simulink model "RIO_DKin_Simul"  (R2024b)
settings: Solver=VariableStepAuto  StartTime=0.0  StopTime=inf  RelTol=1e-3  EnableMultiTasking=on
libraries: vrlib x7, simulink x6, RIO_Lib x1
settings Model: Creator=jorgemartins  LastModifiedBy=pepev
settings SolverCC: AlgebraicLoopSolver=TrustRegion
settings DataIOCC: LimitDataPoints=on  ReturnWorkspaceOutputs=off
settings OptimizationCC: LifeSpan=inf
settings DebuggingCC: UnconnectedInputMsg=warning  UnconnectedOutputMsg=warning  UnconnectedLineMsg=warning  AllowSymbolicDim=off  SFUnexpectedBacktrackingDiag=warning  SFNoUnconditionalDefaultTransitionDiag=warning  SFExecutionAtInitializationDiag=none  ArithmeticOperatorsInVariantConditions=warning
settings ModelReferenceCC: EnableRefExpFcnMdlSchedulingChecks=on  PropagateSignalLabelsOutOfModel=off
settings SFSimCC: SimUseLocalCustomCode=off  CustomCodeUndefinedFunction=UseInterfaceOnly
settings RTWCC: RTWUseLocalCustomCode=off  GPUComputeCapability=3.5
settings CodeAppCC: StateflowObjectComments=on
settings GRTTargetCC: TargetLangStandard=C89/C90 (ANSI)
settings ConfigComp: CovMetricSettings=dw  CovSaveCumulativeToWorkspaceVar=on  CovSaveSingleToWorkspaceVar=on  CovExternalEMLEnable=off

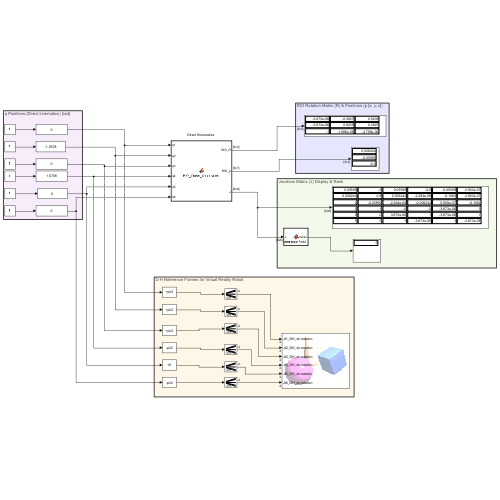
[thumbnail: Simulink's stored preview of the top-level diagram]
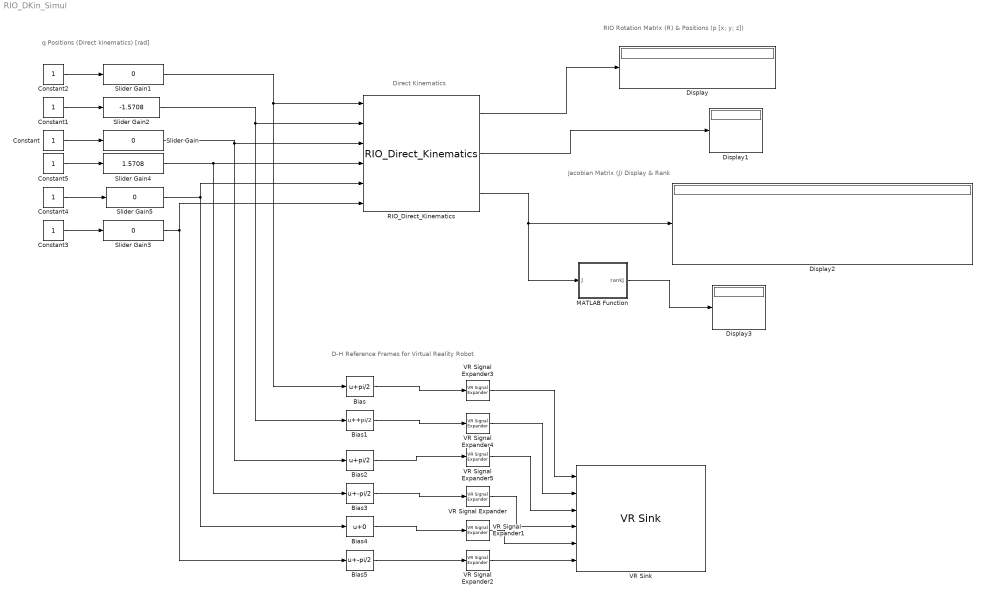
== system RIO_DKin_Simul ==
  note: Direct Kinematics
  note: D-H Reference Frames for Virtual Reality Robot
  note: Jacobian Matrix (J) Display & Rank
  note: RIO Rotation Matrix (R) & Positions (p [x; y; z])
  note: q Positions (Direct kinematics) [rad]
  Bias : Bias  Bias=pi/2  SaturateOnIntegerOverflow=off
  Bias1 : Bias  Bias=+pi/2  SaturateOnIntegerOverflow=off
  Bias2 : Bias  Bias=pi/2  SaturateOnIntegerOverflow=off
  Bias3 : Bias  Bias=-pi/2  SaturateOnIntegerOverflow=off
  Bias4 : Bias  SaturateOnIntegerOverflow=off
  Bias5 : Bias  Bias=-pi/2  SaturateOnIntegerOverflow=off
  Constant{,1..5} (6 alike) : Constant
  Display{,1..3} (4 alike) : Display
  MATLAB Function : MATLAB Function  TreatAsAtomicUnit=on
  RIO_Direct_Kinematics : RIO_Lib/RIO_Direct_Kinematics  SystemSampleTime=-1  VariantActivationTime=update diagram  AllowFlexibleInterface=on  Latency=0  AutoFrameSizeCalculation=off
  Slider Gain{,1,3,5} (4 alike) : simulink/Math Operations/Slider Gain  gain=0  low=-3.14  high=3.14
  Slider Gain2 : simulink/Math Operations/Slider Gain  gain=-1.5708  low=-3.14  high=3.14
  Slider Gain4 : simulink/Math Operations/Slider Gain  gain=1.5708  low=-3.14  high=3.14
  VR Signal Expander{,1..5} (6 alike) : vrlib/VR Signal Expander  outwidth=4  outidx=[4]
  VR Sink : vrlib/VR Sink  InstantiateOnLoad=on  SampleTime=-1  ViewEnable=on  RemoteChange=off  RemoteView=off  FieldsWritten=Jt1_DH_dv.rotation.4.1.1.double#Jt2_DH_dv.rotation.4.1.1.double#Jt3_DH_dv.rotation.4.1.1.double#Jt4_DH_dv.rotation.4.1.1.double#Jt5_DH_dv.rotation.4.1.1.double#Jt6_DH_dv.rotation.4.1.1.double  WorldFileName=vrrobot.wrl  WorldDescription=D-H Reference Frames for Virtual Reality Robot  AutoView=on  VideoDimensions=[]  AllowVariableSize=off
  wires:
  RIO_Direct_Kinematics/1 -> Display/1
  RIO_Direct_Kinematics/2 -> Display1/1
  Constant/1 -> Slider Gain/1
  Slider Gain/1 -> Bias2/1, RIO_Direct_Kinematics/3
  Constant2/1 -> Slider Gain1/1
  Slider Gain1/1 -> Bias/1, RIO_Direct_Kinematics/1
  Constant1/1 -> Slider Gain2/1
  Slider Gain2/1 -> Bias1/1, RIO_Direct_Kinematics/2
  Constant3/1 -> Slider Gain3/1
  Constant4/1 -> Slider Gain5/1
  Constant5/1 -> Slider Gain4/1
  Bias/1 -> VR Signal Expander3/1
  Bias1/1 -> VR Signal Expander4/1
  Bias2/1 -> VR Signal Expander5/1
  Bias3/1 -> VR Signal Expander/1
  Bias4/1 -> VR Signal Expander1/1
  Bias5/1 -> VR Signal Expander2/1
  Slider Gain4/1 -> Bias3/1, RIO_Direct_Kinematics/4
  Slider Gain5/1 -> RIO_Direct_Kinematics/5, Bias4/1
  Slider Gain3/1 -> RIO_Direct_Kinematics/6, Bias5/1
  VR Signal Expander3/1 -> VR Sink/1
  VR Signal Expander4/1 -> VR Sink/2
  VR Signal Expander5/1 -> VR Sink/3
  VR Signal Expander/1 -> VR Sink/4
  VR Signal Expander1/1 -> VR Sink/5
  VR Signal Expander2/1 -> VR Sink/6
  RIO_Direct_Kinematics/3 -> MATLAB Function/1(J), Display2/1
  MATLAB Function/1(rankJ) -> Display3/1

== matlab function RIO_DKin_Simul/MATLAB Function ==
  data: J input double size=[6,6]; rankJ output double size=[1 1]
function rankJ = computeRank(J)
%#codegen
 tol = 1e-4;  % tolerance
 rankJ = rank(J, tol);
end
